simulink model "eml_2nd_order_filter"  (Simulink 7.3)
settings: Solver=FixedStepDiscrete  StartTime=0.0  StopTime=1  RelTol=1e-3
values from neighbouring files (symbols this model uses):
  den = [1.0                0.0                0.171600341796875]    [fi_datatype_override_demo.m]    (also in numbercircle.m = den(ones(size(bin,1),1),:))
  num = [0.29290771484375   0.585784912109375  0.292907714843750]    [fi_datatype_override_demo.m]    (also in numbercircle.m = [bin equiv num2str(x)])
libraries: simulink x1
settings Model: Creator=tbryan  LastModifiedBy=sbatabya  ExtModeAutoUpdateStatusClock=off
settings OptimizationCC: IndividualOutputsThreshold=0  InitFltsAndDblsToZero=on
settings DebuggingCC: SaveWithParameterizedLinksMsg=none  SignalResolutionControl=TryResolveAllWithWarning  MultiTaskDSMMsg=warning  MultiTaskCondExecSysMsg=none  SigSpecEnsureSampleTimeMsg=none  IntegerOverflowMsg=none  Int32ToFloatConvMsg=none  ParameterOverflowMsg=none  ParameterPrecisionLossMsg=none
settings RTWCC: IncludeERTFirstTime=on
settings GRTTargetCC: TargetFcnLib=ansi_tfl_tmw.mat

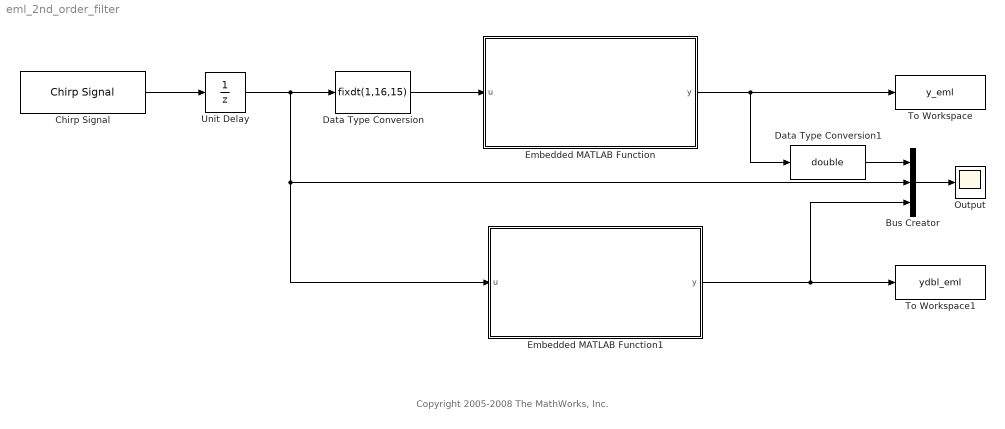
== system eml_2nd_order_filter ==
  note: Copyright 2005-2008 The MathWorks, Inc.
  Bus Creator : BusCreator  Inputs=3
  Chirp Signal : simulink/Sources/Chirp Signal  SystemSampleTime=-1  f1=0  T=1  f2=128
  Data Type Conversion : DataTypeConversion  OutDataTypeMode=Specify via dialog  OutDataType=fixdt(1,16,15)  OutDataTypeStr=fixdt(1,16,15)  RndMeth=Nearest  SaturateOnIntegerOverflow=on
  Data Type Conversion1 : DataTypeConversion  OutDataTypeMode=double  OutDataType=sfix(16)  OutScaling=2^-15  OutDataTypeStr=double  RndMeth=Nearest  SaturateOnIntegerOverflow=on
  Embedded MATLAB Function : Stateflow chart
  Embedded MATLAB Function1 : Stateflow chart
  Output : Scope
      settings: TimeRange=1
  To Workspace : ToWorkspace  VariableName=y_eml  SampleTime=-1  SaveFormat=Array
  To Workspace1 : ToWorkspace  VariableName=ydbl_eml  SampleTime=-1  SaveFormat=Array
  Unit Delay : UnitDelay  SampleTime=1/256
  wires:
  Chirp Signal/1 -> Unit Delay/1
  Data Type Conversion/1 -> Embedded MATLAB Function/1(u)
  Bus Creator/1 -> Output/1
  Embedded MATLAB Function/1(y) -> To Workspace/1, Data Type Conversion1/1
  Unit Delay/1 -> Data Type Conversion/1, Bus Creator/2, Embedded MATLAB Function1/1(u)
  Embedded MATLAB Function1/1(y) -> To Workspace1/1, Bus Creator/3
  Data Type Conversion1/1 -> Bus Creator/1

== matlab function Embedded MATLAB Function1 ==
  data: num parameter double; den parameter double; u input double; y output double
function y = fi_2nd_order_filter(num, den, u)
%   Copyright 2005 The MathWorks, Inc.
%   $Revision: 1.1.6.2 $  $Date: 2008/12/01 07:13:07 $

y = fieml_2nd_order_filter(num, den, u);

== matlab function Embedded MATLAB Function ==
  data: num parameter double; den parameter double; u input double; y output double
function y = fi_2nd_order_filter(num, den, u)
%   Copyright 2005 The MathWorks, Inc.
%   $Revision: 1.1.6.2 $  $Date: 2008/12/01 07:13:07 $

y = fieml_2nd_order_filter(num,den,u);
